simulink model "countertests"  (R2021a)
settings: Solver=VariableStepAuto  StartTime=0.0  StopTime=10.0  RelTol=1e-3
libraries: simulink x1, UtilityLibrary x1
settings Model: Creator=phill  LastModifiedBy=phill

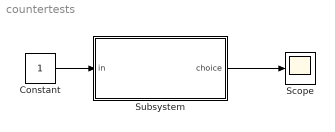
== system countertests ==
  Constant : Constant
  Scope : Scope
  Subsystem : Subsystem  mask{resetThreshold=1}
      mask prompts: resetThreshold "reset threshold"
      mask Display:
      | disp('Cyc Enabler \n\n');
      | disp(['resets at x = ', get_param(gcb,'resetThreshold')])
  wires:
  Constant/1 -> Subsystem/1(in)
  Subsystem/1(choice) -> Scope/1

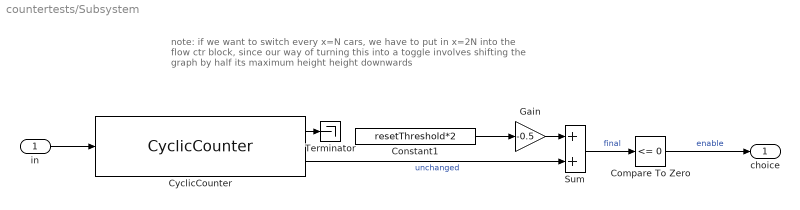
== system countertests/Subsystem ==
  note: note: if we want to switch every x=N cars, we have to put in x=2N
      | into the flow ctr block, since our way of turning this into a toggle involves
      | shifting the graph by half its maximum height height downwards
  in : Inport
  Compare To Zero : simulink/Logic and Bit Operations/Compare To Zero  relop=<=  OutDataTypeStr=boolean
  Constant1 : Constant  Value=resetThreshold*2
  CyclicCounter : UtilityLibrary/CyclicCounter  resetThreshold=resetThreshold*2
  Gain : Gain  Gain=-0.5
  Sum : Sum
  Terminator : Terminator
  choice : Outport
  wires:
  Compare To Zero/1 -> choice/1  "enable"
  in/1 -> CyclicCounter/1
  Sum/1 -> Compare To Zero/1  "final"
  Gain/1 -> Sum/1
  Constant1/1 -> Gain/1
  CyclicCounter/2 -> Sum/2  "unchanged"
  CyclicCounter/1 -> Terminator/1
